simulink model "wheel_speed_generated"  (R2024b)
settings: Solver=VariableStepAuto  StartTime=0.0  StopTime=10.0  RelTol=1e-3
settings Model: Creator=xinxing  LastModifiedBy=xinxing

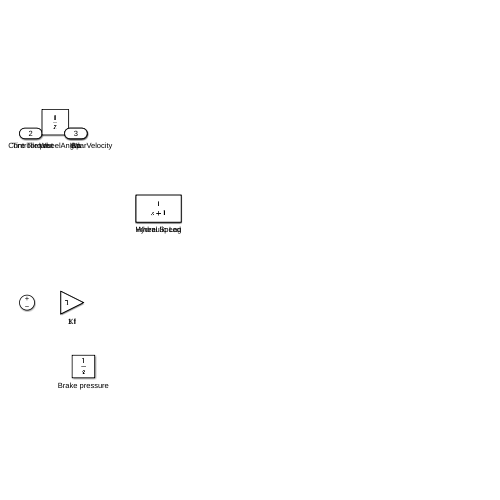
[thumbnail: Simulink's stored preview of the top-level diagram]
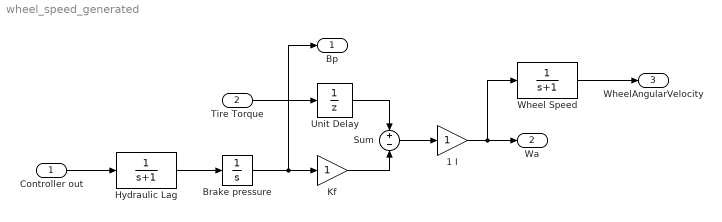
== system wheel_speed_generated ==
  Controller out : Inport
  Tire Torque : Inport  Port=2
  1 I : Gain
  Brake pressure : Integrator
  Hydraulic Lag : TransferFcn  Denominator=[1 1]
  Kf : Gain
  Sum : Sum  Inputs=+-
  Unit Delay : UnitDelay  SampleTime=-1  HasFrameUpgradeWarning=on
  Wheel Speed : TransferFcn  Denominator=[1 1]
  Bp : Outport
  Wa : Outport  Port=2
  WheelAngularVelocity : Outport  Port=3
  wires:
  1 I/1 -> Wa/1, Wheel Speed/1
  Wheel Speed/1 -> WheelAngularVelocity/1
  Sum/1 -> 1 I/1
  Kf/1 -> Sum/2
  Unit Delay/1 -> Sum/1
  Brake pressure/1 -> Bp/1, Kf/1
  Tire Torque/1 -> Unit Delay/1
  Hydraulic Lag/1 -> Brake pressure/1
  Controller out/1 -> Hydraulic Lag/1
